simulink model "modelo_NL_LQRY_GUIA"  (R2025b)
settings: Solver=ode4  StartTime=0.0  StopTime=TimeXP  FixedStep=Ts  RelTol=1e-3
values from neighbouring files (symbols this model uses):
  alpha_prot = deg2rad(16)    [NL_missao_lqry3.m]    (also in XP_missao_lqry3.m)
  att_alt = 0    [NL_missao_lqry3.m]    (also in XP_missao_lqry3.m)
  de_trim = XP_U_trim4(2)    [NL_missao_lqry3.m]    (also in XP_missao_lqry3.m = deg2rad(XP_de0_dg))
  h_ref0 = 600    [NL_missao_lqry3.m]    (also in XP_missao_lqry3.m = XP_h_ref0)
  i = find([Plantas.Ve] == NL3_VT & [Plantas.He] == 600, 1)    [NL_missao_lqry3.m]    (also in XP_missao_lqry3.m = find([Plantas.Ve] == XP3_VT & [Plantas.He] == 600, 1); abre_modelo_NL_LQRY.m = find([Plantas.Ve] == o.VT & [Plantas.He] == 600, 1); arruma_sobreposicoes.m = par(1); lqry_v3_prepara_modelo.m = g('i', evalin('base', 'i')))
  K_bank_guia = 0.1975    [NL_missao_lqry3.m]    (also in XP_missao_lqry3.m)
  phi_max_guia = deg2rad(20)    [NL_missao_lqry3.m]    (also in XP_missao_lqry3.m)
  phi_psi = NL3_phi_psi    [NL_missao_lqry3.m]    (also in XP_missao_lqry3.m = XP3_phi_psi)
  Plantas = S.Plantas; assignin('base', 'Plantas', Plantas)    [abre_modelo_NL_LQRY.m]    (also in tabela_ganhos.m = S.Plantas)
  prot_on = 0    [NL_missao_lqry3.m]    (also in XP_missao_lqry3.m = XP3_prot)
  R_accept = NL3_R_accept    [NL_missao_lqry3.m]    (also in XP_missao_lqry3.m = XP3_R_accept; build_pacote_mirko.m = raio de captura [m].\n'   ')
  refAlt = 0    [NL_missao_lqry3.m]    (also in XP_missao_lqry3.m)
  refPhi = 0    [NL_missao_lqry3.m]    (also in XP_missao_lqry3.m)
  refPsi = 0    [NL_missao_lqry3.m]    (also in XP_missao_lqry3.m)
  reftheta = 0    [NL_missao_lqry3.m]    (also in XP_missao_lqry3.m)
  refVel = NL3_VT    [NL_missao_lqry3.m]    (also in XP_missao_lqry3.m = XP3_VT)
  sat_surf_rad = deg2rad(NL3_sat_deg)    [NL_missao_lqry3.m]
  surfaces = 24    [NL_missao_lqry3.m]    (also in XP_missao_lqry3.m)
  VT_ref0 = NL3_VT    [NL_missao_lqry3.m]    (also in XP_missao_lqry3.m = XP3_VT)
  VT_Throttle = 1    [NL_missao_lqry3.m]    (also in XP_missao_lqry3.m)
  WPs = WPs_user(1,:)    [NL_missao_lqry3.m]    (also in XP_missao_lqry3.m; abre_modelo_NL_LQRY.m = [256 0 600 15; 416 160 600 15; 256 320 600 15; 0 320 600 15;)
  XP_clamp_lqry = deg2rad(NL3_clamp_deg)    [NL_missao_lqry3.m]    (also in XP_missao_lqry3.m = deg2rad(XP3_clamp_deg))
  XP_h_ref0 = 600    [NL_missao_lqry3.m]    (also in XP_missao_lqry3.m = XP_msl0)
  XP_IC_int_alt = 0    [XP_missao_lqry3.m]
  XP_IC_int_speed = 0    [XP_missao_lqry3.m]
  XP_IC_int_theta = 0    [XP_missao_lqry3.m]
  XP_U_trim4 = double(Plantas(i).Ue(1:4))    [NL_missao_lqry3.m]    (also in XP_missao_lqry3.m = [XP_thr0; deg2rad(XP_de0_dg); 0; 0])
undefined symbols (not defined in the file or in its folder): act, eng, TrimInput
libraries: simulink_extras x14
settings Model: SimulationMode=accelerator  Creator=mirko  LastModifiedBy=kaue

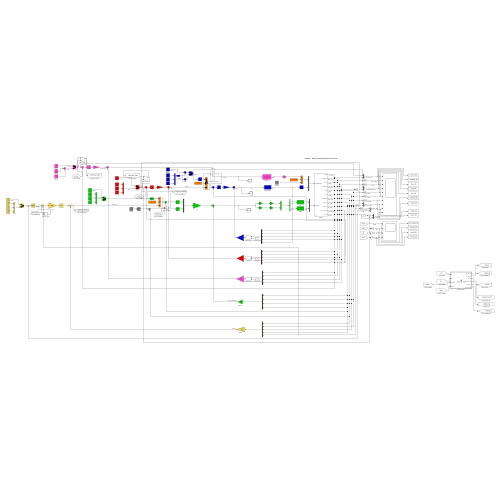
[thumbnail: Simulink's stored preview of the top-level diagram]
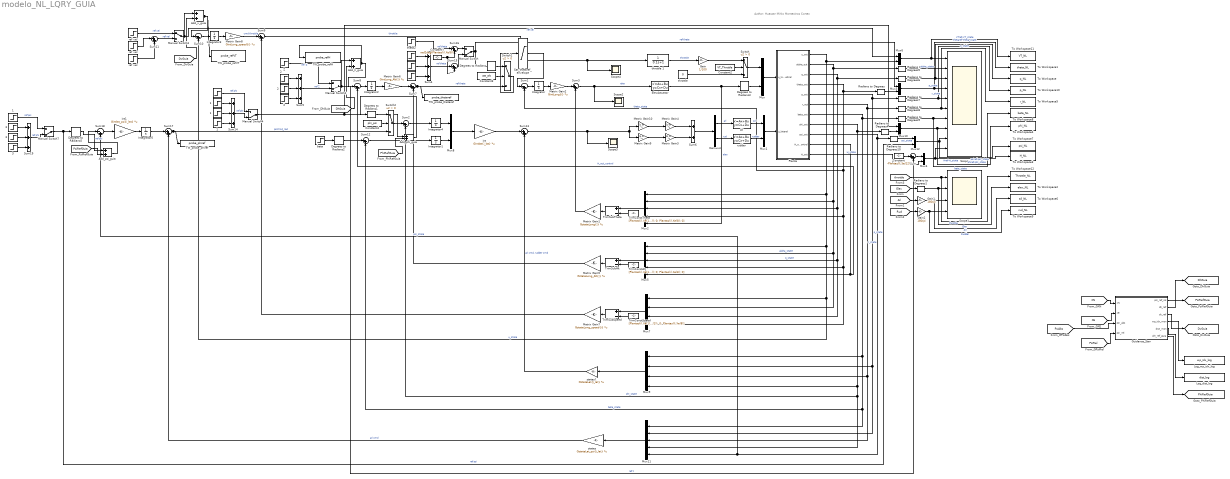
== system modelo_NL_LQRY_GUIA ==
  note: Author: Huascar Mirko Montecinos Cortez
  "   " : Step  Time=80  After=refPhi  SampleTime=0
  "     " : Step  Time=40  After=reftheta  SampleTime=0
  "          " : Step  Time=80  Before=-reftheta  After=0  SampleTime=0
  "            " : Step  Time=60  Before=reftheta  After=-reftheta  SampleTime=0
  "            1" : Step  Time=110  Before=refPhi  After=-refPhi  SampleTime=0
  "            2" : Step  Time=60  Before=refAlt  After=-refAlt  SampleTime=0
  "            3" : Step  Time=110  Before=refPsi  After=-refPsi  SampleTime=0
  "          1" : Step  Time=130  Before=-refPhi  After=0  SampleTime=0
  "          2" : Step  Time=80  Before=-refAlt  After=0  SampleTime=0
  "          3" : Step  Time=130  Before=-refPsi  After=0  SampleTime=0
  "     1" : Step  Time=90  After=refPhi  SampleTime=0
  "     2" : Step  Time=40  After=refAlt  SampleTime=0
  "     3" : Step  Time=90  After=refPsi  SampleTime=0
  "   1" : Step  Time=80  After=refPsi  SampleTime=0
  " Z " : Step  Time=40  After=refAlt  SampleTime=0
  " ref vel " : Step  Time=5  Before=refVel  After=refVel  SampleTime=0
  Add_h_guia : Sum
  Add_phi_guia : Sum
  Add_psi_guia : Sum
  Add_v_guia : Sum
  Ail : StateSpace  A=-surfaces  B=surfaces  D=0  InitialCondition=0
  Constant : Constant  Value=-Plantas(i).Xe(12)
  Constant1 : Constant  Value=rad2deg(Plantas(i).Xe(8))
  Constant2 : Constant  Value=VT_Throttle
  Constant3 : Constant  Value=att_alt
  Constant4 : Constant  Value=phi_psi
  Degrees to Radians{,1..3,5} (5 alike) : simulink_extras/Transformations/Degrees to Radians
  Demux4 : Demux  Outputs=2
      settings: DisplayOption=none
  ElevActuator : StateSpace  A=-surfaces  B=surfaces  D=0  InitialCondition=Plantas(i).Ue(2)
  Gain : Gain  Gain=1/100
  Gain1 : Gain  Gain=180/pi
  Gain2 : Gain  Gain=180/pi
  Guidance_Star : MATLAB Function  TreatAsAtomicUnit=on
  Integrator : Integrator  InitialCondition=XP_IC_int_theta
  Integrator1 : Integrator
  Integrator2 : Integrator  InitialCondition=XP_IC_int_alt
  Integrator3 : Integrator  InitialCondition=XP_IC_int_speed
  Integrator4 : Integrator
  Integrator5 : Integrator
  Log_dist_log : ToWorkspace  VariableName=dist_log  SampleTime=-1
  Log_wp_idx_log : ToWorkspace  VariableName=wp_idx_log  SampleTime=-1
  Manual Switch{,2,4,7} (4 alike) : ManualSwitch  CurrentSetting=0
  Manual Switch3 : ManualSwitch
  Matrix Gain1 : Gain  Gain=GstateLong{i}  Multiplication=Matrix(K*u)  SaturateOnIntegerOverflow=on  OutDataTypeStr=Inherit: Same as input  ParamDataTypeStr=Inherit: Same as input
  Matrix Gain10 : Gain  Gain=[1 0]  Multiplication=Matrix(K*u)  SaturateOnIntegerOverflow=on  OutDataTypeStr=Inherit: Same as input  ParamDataTypeStr=Inherit: Same as input
  Matrix Gain2 : Gain  Gain=GintLong{i}  Multiplication=Matrix(K*u)  SaturateOnIntegerOverflow=on  OutDataTypeStr=Inherit: Same as input  ParamDataTypeStr=Inherit: Same as input
  Matrix Gain3 : Gain  Gain=[0 1]'  Multiplication=Matrix(K*u)  SaturateOnIntegerOverflow=on  OutDataTypeStr=Inherit: Same as input  ParamDataTypeStr=Inherit: Same as input
  Matrix Gain4 : Gain  Gain=[1 0]'  Multiplication=Matrix(K*u)  SaturateOnIntegerOverflow=on  OutDataTypeStr=Inherit: Same as input  ParamDataTypeStr=Inherit: Same as input
  Matrix Gain5 : Gain  Gain=GstateLong_Alt{i}  Multiplication=Matrix(K*u)  SaturateOnIntegerOverflow=on  OutDataTypeStr=Inherit: Same as input  ParamDataTypeStr=Inherit: Same as input
  Matrix Gain6 : Gain  Gain=GintLong_Alt{i}  Multiplication=Matrix(K*u)  SaturateOnIntegerOverflow=on  OutDataTypeStr=Inherit: Same as input  ParamDataTypeStr=Inherit: Same as input
  Matrix Gain7 : Gain  Gain=GstateLong_speed{i}  Multiplication=Matrix(K*u)  SaturateOnIntegerOverflow=on  OutDataTypeStr=Inherit: Same as input  ParamDataTypeStr=Inherit: Same as input
  Matrix Gain8 : Gain  Gain=GintLong_speed{i}  Multiplication=Matrix(K*u)  SaturateOnIntegerOverflow=on  OutDataTypeStr=Inherit: Same as input  ParamDataTypeStr=Inherit: Same as input
  Matrix Gain9 : Gain  Gain=[0 1]  Multiplication=Matrix(K*u)  SaturateOnIntegerOverflow=on  OutDataTypeStr=Inherit: Same as input  ParamDataTypeStr=Inherit: Same as input
  Mux{,1,3..4,6,8,10,12} (8 alike) : Mux  Inputs=2
  Mux11 : Mux  Inputs=5
  Mux2 : Mux  Inputs=5
  Mux5 : Mux  Inputs=5
  Mux7 : Mux
  Mux9 : Mux
  Planta : Subsystem
  Radians to Degrees{,1,4..10} (9 alike) : simulink_extras/Transformations/Radians to Degrees
  Sat_thetaref_envelope : Saturate  UpperLimit=XP_clamp_lqry(2)  LowerLimit=XP_clamp_lqry(1)
  Scope : Scope  NumInputPorts=10
      settings: ActiveDisplayString=10  ActiveDisplayYMinimum=593.67577098481627  ActiveDisplayYMaximum=606.307142927377
  Scope1 : Scope  NumInputPorts=4
      settings: ActiveDisplayString=4  ActiveDisplayYMinimum=-3.1238215479894382  ActiveDisplayYMaximum=4.435550961328742
  Scope2 : Scope
      settings: ActiveDisplayYMinimum=-1.3531942213324573  ActiveDisplayYMaximum=0.61662907005096645  DataLoggingVariableName=ScopeData2
  Scope3 : Scope
      settings: ActiveDisplayYMinimum=-0.008953837623387962  ActiveDisplayYMaximum=0.0080763644870395709  DataLoggingVariableName=ScopeData3
  Scope4 : Scope
      settings: ActiveDisplayYMinimum=-268.65761065429206  ActiveDisplayYMaximum=1519.894817061396  DataLoggingVariableName=ScopeData4
  Sum{,3,7,9,11,15..16} (7 alike) : Sum  Inputs=|++
  Sum1 : Sum  Inputs=|-+
  Sum10 : Sum  Inputs=|-+
  Sum12 : Sum  Inputs=|-+  SaturateOnIntegerOverflow=on
  Sum13 : Sum  Inputs=|++  SaturateOnIntegerOverflow=on
  Sum{4..5,14,19} (4 alike) : Sum  Inputs=+++
  Sum17 : Sum  Inputs=|++  SaturateOnIntegerOverflow=on
  Sum18 : Sum  Inputs=|-+  SaturateOnIntegerOverflow=on
  Sum2 : Sum  Inputs=|-+  SaturateOnIntegerOverflow=on
  Sum6 : Sum  Inputs=2  SaturateOnIntegerOverflow=on
  Sum8 : Sum  Inputs=|-+
  Switch : Switch  Criteria=u2 > Threshold  SaturateOnIntegerOverflow=off  InputSameDT=off
  Switch1 : Switch  Criteria=u2 > Threshold  SaturateOnIntegerOverflow=off  InputSameDT=off
  Switch2 : Switch  Criteria=u2 > Threshold  SaturateOnIntegerOverflow=off  InputSameDT=off
  TW_probe_phiref : ToWorkspace  VariableName=probe_phiref  SampleTime=-1
  TW_probe_refH : ToWorkspace  VariableName=probe_refH  SampleTime=-1
  TW_probe_refVT : ToWorkspace  VariableName=probe_refVT  SampleTime=-1
  TW_probe_thetaref : ToWorkspace  VariableName=probe_thetaref  SampleTime=-1
  To Workspace : ToWorkspace  VariableName=q_NL  SaveFormat=Structure With Time  SampleTime=-1
  To Workspace1 : ToWorkspace  VariableName=theta_NL  SaveFormat=Structure With Time  SampleTime=-1
  To Workspace10 : ToWorkspace  VariableName=p_NL  SaveFormat=Structure With Time  SampleTime=-1
  To Workspace11 : ToWorkspace  VariableName=VT_NL  SaveFormat=Structure With Time  SampleTime=-1
  To Workspace12 : ToWorkspace  VariableName=Throttle_NL  SaveFormat=Structure With Time  SampleTime=-1
  To Workspace2 : ToWorkspace  VariableName=elev_NL  SaveFormat=Structure With Time  SampleTime=-1
  To Workspace3 : ToWorkspace  VariableName=H_NL  SaveFormat=Structure With Time  SampleTime=-1
  To Workspace4 : ToWorkspace  VariableName=phi_NL  SaveFormat=Structure With Time  SampleTime=-1
  To Workspace5 : ToWorkspace  VariableName=r_NL  SaveFormat=Structure With Time  SampleTime=-1
  To Workspace6 : ToWorkspace  VariableName=ail_NL  SaveFormat=Structure With Time  SampleTime=-1
  To Workspace7 : ToWorkspace  VariableName=psi_NL  SaveFormat=Structure With Time  SampleTime=-1
  To Workspace8 : ToWorkspace  VariableName=beta_NL  SaveFormat=Structure With Time  SampleTime=-1
  To Workspace9 : ToWorkspace  VariableName=rud_NL  SaveFormat=Structure With Time  SampleTime=-1
  TrimConstAlt : Constant  Value=[Plantas(i).Xe(1); atan(Plantas(i).Xe(3)/Plantas(i).Xe(1)); 0; Plantas(i).Xe(8); 0]  VectorParams1D=off
  TrimConstSpeed : Constant  Value=[Plantas(i).Xe(1); atan(Plantas(i).Xe(3)/Plantas(i).Xe(1)); 0; Plantas(i).Xe(8)]  VectorParams1D=off
  TrimConstTheta : Constant  Value=[Plantas(i).Xe(1); atan(Plantas(i).Xe(3)/Plantas(i).Xe(1)); 0; Plantas(i).Xe(8); 0]  VectorParams1D=off
  TrimSubAlt : Sum  Inputs=+-
  TrimSubSpeed : Sum  Inputs=+-
  TrimSubTheta : Sum  Inputs=+-
  beta : Step  Time=0  After=0  SampleTime=0
  int : Gain  Gain=Gintlat{i_lat}  Multiplication=Matrix(K*u)  SaturateOnIntegerOverflow=on  OutDataTypeStr=Inherit: Same as input  ParamDataTypeStr=Inherit: Same as input
  int1 : Gain  Gain=Gintlat_psi{i_lat}  Multiplication=Matrix(K*u)  SaturateOnIntegerOverflow=on  OutDataTypeStr=Inherit: Same as input  ParamDataTypeStr=Inherit: Same as input
  ref vel : Step  Time=10  Before=Plantas(i).Xe(1)  After=Plantas(i).Xe(1)+3  SampleTime=0
  "ref vel  " : Step  Time=20  After=-3  SampleTime=0
  rudder : StateSpace  A=-surfaces  B=surfaces  D=0  InitialCondition=0
  states : Gain  Gain=GstateLat_psi{i_lat}  Multiplication=Matrix(K*u)  SaturateOnIntegerOverflow=on  OutDataTypeStr=Inherit: Same as input  ParamDataTypeStr=Inherit: Same as input
  states1 : Gain  Gain=GstateLat{i_lat}  Multiplication=Matrix(K*u)  SaturateOnIntegerOverflow=on  OutDataTypeStr=Inherit: Same as input  ParamDataTypeStr=Inherit: Same as input
  theta2 : Step  Time=100  After=reftheta  SampleTime=0
  throttle : Constant  Value=0
  throttle 1 : TransferFcn  Denominator=[0.1 1]
  tag scope: DhGuia=global, DvGuia=global, PhiRefGuia=global, PsiRefGuia=global
  wires:
  Mux/1 -> Planta/1(u_longitudinal)
  Mux1/1 -> Planta/2(u_lateral)
  Manual Switch/1 -> Degrees to Radians/1, Mux3/1  "ref theta"
  Matrix Gain1/1 -> Sum3/2
  Matrix Gain2/1 -> Sum3/1
  Integrator/1 -> Matrix Gain2/1
  Sum4/1 -> Sum15/1  "ref theta"
  Sum1/1 -> Integrator/1
  theta2/1 -> Sum16/1  "ref theta"
  Sum3/1 -> Scope2/1, ElevActuator/1  "elev"
  Planta/1(u_out) -> Mux6/2, Mux7/1, Sum10/2, Mux5/1, Mux2/1  "u_state"
  Planta/2(alpha_out) -> Mux7/2, Mux5/2, Mux2/2, Radians to Degrees5/1  "alpha_state"
  Planta/3(q_out) -> Mux7/3, Mux5/3, Mux2/3, Radians to Degrees6/1  "q_state"
  Planta/4(theta_out) -> Mux7/4, Mux5/4, Mux2/4, Sum1/2, Radians to Degrees/1  "theta_state"
  Planta/5(p_out) -> Radians to Degrees7/1, Mux9/2, Mux11/2  "p_state"
  Planta/6(r_out) -> Radians to Degrees8/1, Mux9/3, Mux11/3  "r_state"
  Planta/7(beta_out) -> Radians to Degrees9/1, Mux11/1, Sum12/2, Mux9/1  "beta_state"
  Planta/8(phi_out) -> Radians to Degrees4/1, Mux11/4, Sum2/2, Mux9/4  "phi_state"
  Planta/9(psi_out) -> Mux11/5, Sum18/2, Radians to Degrees10/1  "psi_state"
  Planta/10(H_out_control) -> Mux5/5, Sum8/2  "H_out_control"
  Mux3/1 -> To Workspace1/1, Scope/4  "thetaref-theta_state"
  Radians to Degrees/1 -> Mux3/2
  Matrix Gain5/1 -> Sum7/2
  " Z "/1 -> Manual Switch2/1  "ref  Z"
  Manual Switch2/1 -> Sum/2, Add_h_guia/1  "ref z"
  Sum8/1 -> Integrator2/1
  Sum7/1 -> Switch1/3, TW_probe_thetaref/1  "ref theta"
  Sum5/1 -> Manual Switch2/2  "ref Z"
  Matrix Gain6/1 -> Sum7/1
  Integrator2/1 -> Matrix Gain6/1
  Degrees to Radians/1 -> Switch1/1
  Mux4/1 -> Scope/10, To Workspace3/1  "Href-H_state"
  Constant/1 -> Sum/1
  Sum/1 -> Mux4/1
  Radians to Degrees1/1 -> Scope1/2, To Workspace2/1  "Elev"
  Gain1/1 -> Scope1/3, To Workspace6/1  "Ail"
  Gain2/1 -> Scope1/4, To Workspace9/1  "Rudder"
  "ref vel  "/1 -> Sum11/2
  Sum10/1 -> Integrator3/1
  ref vel/1 -> Sum11/1
  Matrix Gain7/1 -> Sum9/2
  " ref vel "/1 -> Manual Switch3/1  "ref vel"
  Manual Switch3/1 -> Mux6/1, Add_v_guia/1  "ref vel"
  Integrator3/1 -> Matrix Gain8/1
  Sum11/1 -> Manual Switch3/2  "ref vel"
  Matrix Gain8/1 -> Sum9/1  "cmd throttle"
  [Elev] -> Radians to Degrees1/1
  [Ail] -> Gain1/1
  [Rud] -> Gain2/1
  [throttle] -> To Workspace12/1, Scope1/1  "throttle"
  Sum9/1 -> Scope4/1, throttle 1/1  "throttle"
  Mux6/1 -> To Workspace11/1, Scope/1  "VTref-VT_state"
  Matrix Gain9/1 -> Matrix Gain3/1
  Matrix Gain10/1 -> Matrix Gain4/1
  Matrix Gain4/1 -> Sum6/1
  Sum13/1 -> Scope3/1, Matrix Gain9/1, Matrix Gain10/1
  Matrix Gain3/1 -> Sum6/2
  Sum6/1 -> Demux4/1
  Demux4/2 -> rudder/1  "rud"
  Demux4/1 -> Ail/1  "ail"
  beta/1 -> Degrees to Radians2/1
  "   "/1 -> Manual Switch4/1  "ref phi"
  int/1 -> Sum13/1
  Degrees to Radians2/1 -> Sum12/1
  Mux8/1 -> int/1
  Sum12/1 -> Integrator1/1
  "     1"/1 -> Sum14/1
  Sum14/1 -> Manual Switch4/2  "ref phi"
  "            1"/1 -> Sum14/2
  "          1"/1 -> Sum14/3
  Integrator4/1 -> Mux8/1
  Integrator1/1 -> Mux8/2
  Sum2/1 -> Integrator4/1
  Mux9/1 -> states1/1
  states1/1 -> Sum13/2  "ail cmd, rudder cmd"
  Mux10/1 -> To Workspace4/1, Scope/8  "phiref-phi_state"
  Radians to Degrees4/1 -> Mux10/2
  Manual Switch4/1 -> Mux10/1, Degrees to Radians1/1
  throttle/1 -> Switch/3
  Radians to Degrees5/1 -> Scope/2  "alpha_state"
  Radians to Degrees6/1 -> To Workspace/1, Scope/3  "q_state"
  Radians to Degrees7/1 -> To Workspace10/1, Scope/5  "p_state"
  Radians to Degrees8/1 -> Scope/6, To Workspace5/1  "r_state"
  Radians to Degrees9/1 -> Scope/7, To Workspace8/1  "beta_state"
  Degrees to Radians3/1 -> Mux/2
  Gain/1 -> Switch/1
  Mux12/1 -> To Workspace7/1, Scope/9  "psiref-psi_state"
  Planta/11(H_out) -> Mux4/2  "H_state"
  Constant1/1 -> Sum15/2, Sum16/2
  Sum15/1 -> Manual Switch/2
  Sum16/1 -> Manual Switch/1
  "          "/1 -> Sum4/3
  "     "/1 -> Sum4/1
  "            "/1 -> Sum4/2
  "          2"/1 -> Sum5/3
  "            2"/1 -> Sum5/2
  "     2"/1 -> Sum5/1
  Mux11/1 -> states/1
  Sum18/1 -> int1/1
  Integrator5/1 -> Sum17/1
  Manual Switch7/1 -> Degrees to Radians5/1, Mux12/2  "ref psi"
  int1/1 -> Integrator5/1
  Sum17/1 -> Switch2/3, TW_probe_phiref/1  "psiCmd_rad"
  states/1 -> Sum17/2  "ail cmd"
  Switch2/1 -> Sum2/1
  "     3"/1 -> Sum19/1
  "            3"/1 -> Sum19/2
  "   1"/1 -> Manual Switch7/1  "ref psi"
  Sum19/1 -> Manual Switch7/2  "ref phi"
  "          3"/1 -> Sum19/3
  Radians to Degrees10/1 -> Mux12/1  "psi_state"
  Constant2/1 -> Switch/2
  Constant3/1 -> Switch1/2
  Constant4/1 -> Switch2/2
  Mux7/1 -> TrimSubSpeed/1
  TrimConstSpeed/1 -> TrimSubSpeed/2
  TrimSubSpeed/1 -> Matrix Gain7/1
  Mux2/1 -> TrimSubTheta/1
  TrimConstTheta/1 -> TrimSubTheta/2
  TrimSubTheta/1 -> Matrix Gain1/1
  Mux5/1 -> TrimSubAlt/1
  TrimConstAlt/1 -> TrimSubAlt/2
  TrimSubAlt/1 -> Matrix Gain5/1
  throttle 1/1 -> Gain/1  "throttle"
  rudder/1 -> Mux1/2  "rudder"
  Ail/1 -> Mux1/1  "Ail"
  ElevActuator/1 -> Degrees to Radians3/1, Mux2/5  "elev"
  Switch/1 -> Mux/1
  [XN] -> Guidance_Star/1(xN)
  [PsiRel] -> Guidance_Star/4(psi_rel)
  Guidance_Star/1(psi_ref_rel) -> [PsiRefGuia]
  Guidance_Star/3(dv_ref) -> [DvGuia]
  Guidance_Star/4(wp_idx_mon) -> Log_wp_idx_log/1
  Guidance_Star/5(dist_mon) -> Log_dist_log/1
  Guidance_Star/6(phi_ref_guia) -> [PhiRefGuia]
  Add_h_guia/1 -> Sum8/1, TW_probe_refH/1
  Degrees to Radians1/1 -> Add_phi_guia/1
  Add_phi_guia/1 -> Switch2/1
  Degrees to Radians5/1 -> Add_psi_guia/1  "ref psi"
  [PsiRefGuia] -> Add_psi_guia/2
  Add_psi_guia/1 -> Sum18/1
  Add_v_guia/1 -> Sum10/1, TW_probe_refVT/1
  [PhiRefGuia] -> Add_phi_guia/2
  [DhGuia] -> Add_h_guia/2
  [DvGuia] -> Add_v_guia/2
  [PsiAbs] -> Guidance_Star/3(psi_abs)
  [XE] -> Guidance_Star/2(xE)
  Guidance_Star/2(dh_ref) -> [DhGuia]
  Switch1/1 -> Sat_thetaref_envelope/1
  Sat_thetaref_envelope/1 -> Sum1/1

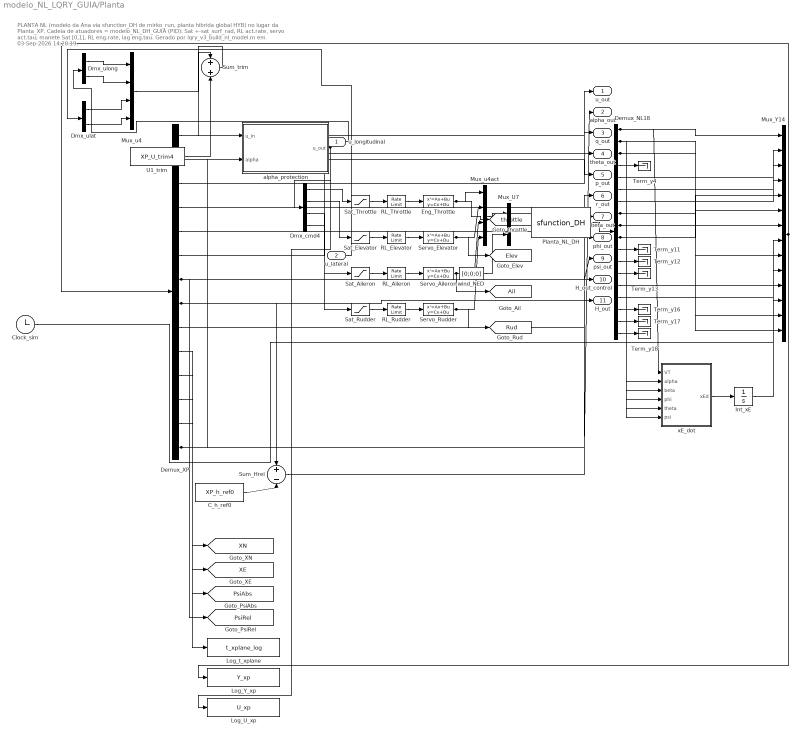
== system modelo_NL_LQRY_GUIA/Planta ==
  note: PLANTA NL (modelo da Ana via sfunction_DH de mirko_run, planta hibrida global HYB)
      | no lugar da Planta_XP. Cadeia de atuadores = modelo_NL_DH_GUIA (PID): Sat +-sat_surf_rad, RL act.rate,
      | servo act.tau; manete Sat [0,1], RL eng.rate, lag eng.tau. Gerado por lqry_v3_build_nl_model.m em 03-Sep-2026 14:20:19.
  u_longitudinal : Inport
  u_lateral : Inport  Port=2
  C_h_ref0 : Constant  Value=XP_h_ref0
  Clock_sim : Clock
  Demux_NL18 : Demux  Outputs=18
  Demux_XP : Demux  Outputs=14
  Dmx_cmd4 : Demux
  Dmx_ulat : Demux  Outputs=2
  Dmx_ulong : Demux  Outputs=2
  Eng_Throttle : StateSpace  A=-1/eng.tau  B=1/eng.tau  D=0  InitialCondition=XP_U_trim4(1)
  Int_xE : Integrator
  Log_U_xp : ToWorkspace  VariableName=U_xp  SampleTime=-1
  Log_Y_xp : ToWorkspace  VariableName=Y_xp  SampleTime=-1
  Log_t_xplane : ToWorkspace  VariableName=t_xplane_log  SampleTime=-1
  Mux_U7 : Mux  Inputs=2
  Mux_Y14 : Mux  Inputs=14
  Mux_u4 : Mux
  Mux_u4act : Mux
  Planta_NL_DH : S-Function  FunctionName=sfunction_DH  Parameters=Xe_planta, coef_Sato, coef_Ana, Variacao_Iner  SFunctionDeploymentMode=off  EnableBusSupport=off
  RL_Aileron : RateLimiter  RisingSlewLimit=act.rate  FallingSlewLimit=-act.rate  InitialCondition=TrimInput(3)
  RL_Elevator : RateLimiter  RisingSlewLimit=act.rate  FallingSlewLimit=-act.rate  InitialCondition=TrimInput(2)
  RL_Rudder : RateLimiter  RisingSlewLimit=act.rate  FallingSlewLimit=-act.rate  InitialCondition=TrimInput(4)
  RL_Throttle : RateLimiter  RisingSlewLimit=eng.rate  FallingSlewLimit=-eng.rate  InitialCondition=TrimInput(1)
  Sat_Aileron : Saturate  UpperLimit=sat_surf_rad  LowerLimit=-sat_surf_rad
  Sat_Elevator : Saturate  UpperLimit=sat_surf_rad  LowerLimit=-sat_surf_rad
  Sat_Rudder : Saturate  UpperLimit=sat_surf_rad  LowerLimit=-sat_surf_rad
  Sat_Throttle : Saturate  UpperLimit=1  LowerLimit=0
  Servo_Aileron : StateSpace  A=-act.bw  B=act.bw  D=0  InitialCondition=XP_U_trim4(3)
  Servo_Elevator : StateSpace  A=-act.bw  B=act.bw  D=0  InitialCondition=XP_U_trim4(2)
  Servo_Rudder : StateSpace  A=-act.bw  B=act.bw  D=0  InitialCondition=XP_U_trim4(4)
  Sum_Hrel : Sum  Inputs=+-
  Sum_trim : Sum
  Term_y{4,11..13,16..18} (7 alike) : Terminator
  U1_trim : Constant  Value=XP_U_trim4
  alpha_protection : MATLAB Function  TreatAsAtomicUnit=on
  wind_NED : Constant  Value=[0;0;0]
  xE_dot : MATLAB Function  TreatAsAtomicUnit=on
  u_out : Outport
  alpha_out : Outport  Port=2
  q_out : Outport  Port=3
  theta_out : Outport  Port=4
  p_out : Outport  Port=5
  r_out : Outport  Port=6
  beta_out : Outport  Port=7
  phi_out : Outport  Port=8
  psi_out : Outport  Port=9
  H_out_control : Outport  Port=10
  H_out : Outport  Port=11
  tag scope: Ail=global, Elev=global, PsiAbs=global, PsiRel=global, Rud=global, XE=global, XN=global, throttle=global
  wires:
  u_longitudinal/1 -> Dmx_ulong/1
  u_lateral/1 -> Dmx_ulat/1
  Dmx_ulong/1 -> Mux_u4/1
  Dmx_ulong/2 -> Mux_u4/2
  Dmx_ulat/1 -> Mux_u4/3
  Dmx_ulat/2 -> Mux_u4/4
  Demux_XP/1 -> u_out/1
  Demux_XP/14 -> alpha_out/1, alpha_protection/2(alpha)
  Demux_XP/3 -> q_out/1
  Demux_XP/6 -> theta_out/1
  Demux_XP/2 -> p_out/1
  Demux_XP/4 -> r_out/1
  Demux_XP/9 -> beta_out/1
  Demux_XP/5 -> phi_out/1
  Demux_XP/7 -> psi_out/1, [PsiRel]
  Demux_XP/8 -> Sum_Hrel/1, H_out/1
  C_h_ref0/1 -> Sum_Hrel/2
  Sum_Hrel/1 -> H_out_control/1
  Demux_XP/11 -> [XN]
  Demux_XP/12 -> [XE]
  Demux_XP/13 -> [PsiAbs]
  Demux_XP/10 -> Log_t_xplane/1
  Mux_u4/1 -> Sum_trim/1
  U1_trim/1 -> Sum_trim/2
  Sum_trim/1 -> alpha_protection/1(u_in)
  alpha_protection/1(u_out) -> Log_U_xp/1, Dmx_cmd4/1
  Dmx_cmd4/1 -> Sat_Throttle/1
  Sat_Throttle/1 -> RL_Throttle/1
  RL_Throttle/1 -> Eng_Throttle/1
  Dmx_cmd4/2 -> Sat_Elevator/1
  Sat_Elevator/1 -> RL_Elevator/1
  RL_Elevator/1 -> Servo_Elevator/1
  Dmx_cmd4/3 -> Sat_Aileron/1
  Sat_Aileron/1 -> RL_Aileron/1
  RL_Aileron/1 -> Servo_Aileron/1
  Dmx_cmd4/4 -> Sat_Rudder/1
  Sat_Rudder/1 -> RL_Rudder/1
  RL_Rudder/1 -> Servo_Rudder/1
  Eng_Throttle/1 -> Mux_u4act/1, [throttle]
  Servo_Elevator/1 -> Mux_u4act/2, [Elev]
  Servo_Aileron/1 -> Mux_u4act/3, [Ail]
  Servo_Rudder/1 -> Mux_u4act/4, [Rud]
  Mux_u4act/1 -> Mux_U7/1
  wind_NED/1 -> Mux_U7/2
  Mux_U7/1 -> Planta_NL_DH/1
  Planta_NL_DH/1 -> Demux_NL18/1
  Demux_NL18/4 -> Term_y4/1
  Demux_NL18/11 -> Term_y11/1
  Demux_NL18/12 -> Term_y12/1
  Demux_NL18/13 -> Term_y13/1
  Demux_NL18/16 -> Term_y16/1
  Demux_NL18/17 -> Term_y17/1
  Demux_NL18/18 -> Term_y18/1
  Demux_NL18/1 -> xE_dot/1(VT), Mux_Y14/1
  Demux_NL18/2 -> xE_dot/2(alpha), Mux_Y14/14
  Demux_NL18/3 -> xE_dot/3(beta), Mux_Y14/9
  Demux_NL18/8 -> xE_dot/4(phi), Mux_Y14/5
  Demux_NL18/9 -> xE_dot/5(theta), Mux_Y14/6
  Demux_NL18/10 -> xE_dot/6(psi), Mux_Y14/7, Mux_Y14/13
  xE_dot/1(xEd) -> Int_xE/1
  Demux_NL18/5 -> Mux_Y14/2
  Demux_NL18/6 -> Mux_Y14/3
  Demux_NL18/7 -> Mux_Y14/4
  Demux_NL18/15 -> Mux_Y14/8
  Clock_sim/1 -> Mux_Y14/10
  Demux_NL18/14 -> Mux_Y14/11
  Int_xE/1 -> Mux_Y14/12
  Mux_Y14/1 -> Demux_XP/1, Log_Y_xp/1

== matlab function modelo_NL_LQRY_GUIA/Planta/xE_dot ==
  data: VT input; xEd output; alpha input; beta input; phi input; theta input; psi input
function xEd = xE_dot(VT, alpha, beta, phi, theta, psi)
% velocidade Leste inercial reconstruida das saidas do observador
% (exato p/ vento zero): [u v w] do triedro aerodinamico -> Lnb linha 2.
u = VT*cos(alpha)*cos(beta); v = VT*sin(beta); w = VT*sin(alpha)*cos(beta);
xEd = (sin(phi)*sin(theta)*sin(psi)+cos(phi)*cos(psi))*v ...
    + (cos(phi)*sin(theta)*sin(psi)-sin(phi)*cos(psi))*w ...
    + cos(theta)*sin(psi)*u;
end

== matlab function modelo_NL_LQRY_GUIA/Guidance_Star ==
  settings: updateMethod=DISCRETE  sampleTime=0.05
  data: xN input; psi_ref_rel output; xE input; psi_abs input; psi_rel input; dh_ref output; dv_ref output; wp_idx_mon output; dist_mon output; phi_ref_guia output; WPs parameter; R_accept parameter; h_ref0 parameter; VT_ref0 parameter; K_bank_guia parameter; phi_max_guia parameter
function [psi_ref_rel, dh_ref, dv_ref, wp_idx_mon, dist_mon, phi_ref_guia] = Guidance_Star(xN, xE, psi_abs, psi_rel, WPs, R_accept, h_ref0, VT_ref0, K_bank_guia, phi_max_guia)
% Guiagem LOS por waypoints — versao LQRY (2026-08-30).
% Igual a do PID (chart_44 do Julio adaptado) MAIS a lei bank-to-turn:
% o heading hold do LQRY (phi_psi=0) e' instavel ate no SIL original
% (phi(0)=3 deg -> NaN), entao a guiagem comanda phi_ref DIRETO no
% bank hold nativo (phi_psi=1, o modo validado do artigo):
%   phi_ref = sat(K_bank_guia * wrap(psi_los - psi_abs), +-phi_max_guia)
% com K_bank_guia = V/(g*tau_psi) = 0.1975 (tau_psi=6 s a 12 m/s) — a
% MESMA agressividade de curva do K_heading do PID (comparacao justa;
% a diferenca e' onde a lei mora: no PID dentro do controlador, no
% LQRY na camada de guiagem). Apos capturar o ULTIMO WP: phi_ref=0
% (asas niveladas ate o tempo esgotar).
persistent wp_idx hold_fim
if isempty(wp_idx), wp_idx = 1; hold_fim = 0; end
num_wps = size(WPs, 1);
if wp_idx > num_wps, wp_idx = num_wps; end
dist = sqrt((WPs(wp_idx,1) - xN)^2 + (WPs(wp_idx,2) - xE)^2);
if (dist <= R_accept)
    if wp_idx < num_wps
        wp_idx = wp_idx + 1;
    else
        hold_fim = 1;
    end
end
tN = WPs(wp_idx, 1);
tE = WPs(wp_idx, 2);
psi_los = atan2(tE - xE, tN - xN);
dpsi = mod(psi_los - psi_abs + pi, 2*pi) - pi;
psi_ref_rel = psi_rel + dpsi;   % mantido p/ compat/log (inerte c/ phi_psi=1)
if hold_fim
    phi_ref_guia = 0;
else
    phi_ref_guia = min(max(K_bank_guia*dpsi, -phi_max_guia), phi_max_guia);
end
dh_ref = WPs(wp_idx, 3) - h_ref0;
dv_ref = WPs(wp_idx, 4) - VT_ref0;
wp_idx_mon = wp_idx;
dist_mon = dist;
end

== matlab function modelo_NL_LQRY_GUIA/Planta/alpha_protection ==
  settings: updateMethod=DISCRETE  sampleTime=0.05
  data: u_in input; u_out output; alpha input; prot_on parameter; alpha_prot parameter; de_trim parameter
function u_out = alpha_protection(u_in, alpha, prot_on, alpha_prot, de_trim)
% PROTECAO DE ENVELOPE DA PLATAFORMA (estilo fly-by-wire, 2026-08-30):
% quando alpha medido excede alpha_prot, o teto NOSE-UP do profundor
% desce em rampa (2 deg de alpha) ate o valor de trim — impede
% fisicamente a incursao de estol INDEPENDENTE do controlador.
% Implementada na Planta_XP (a "aeronave"), nao no controlador do
% Mirko: e' o unico jeito efetivo num regulador de estados (o clamp
% de referencia e' contornado pela realimentacao direta — testado).
u_out = u_in;
if prot_on > 0.5
    rampa = 2*pi/180;
    de_max_full = 25*pi/180;
    folga = alpha_prot - alpha;                % >0 abaixo do limite
    frac = min(1, max(0, folga/rampa));        % 1 = livre, 0 = so trim
    de_teto = de_trim + frac*(de_max_full - de_trim);
    u_out(2) = min(u_in(2), de_teto);
end
end
